simulink model "ex1sf"  (Simulink 7.9)
settings: Solver=ode45  StartTime=0.0  StopTime=10.0  RelTol=1e-3
settings Model: Creator=Daniel  LastModifiedBy=Daniel

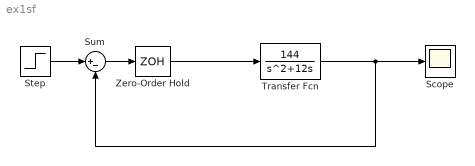
== system ex1sf ==
  Scope : Scope
      settings: TimeRange=10
  Step : Step  Time=0.1  SampleTime=0
  Sum : Sum  Inputs=|+-
  Transfer Fcn : TransferFcn  Numerator=[144]  Denominator=[1 12 0]
  Zero-Order Hold : ZeroOrderHold
  wires:
  Transfer Fcn/1 -> Scope/1, Sum/2
  Zero-Order Hold/1 -> Transfer Fcn/1
  Sum/1 -> Zero-Order Hold/1
  Step/1 -> Sum/1
